simulink model "gm_UZ_D_GaN_Inverter_reduced"  (R2020b)
settings: Solver=FixedStepDiscrete  StartTime=0.0  StopTime=300e-6  RelTol=1e-3
libraries: simulink x24, hdlsllib x6
settings Model: Creator=Michael Hoerner  LastModifiedBy=micha
settings DataIOCC: LimitDataPoints=on  SaveOutput=off  SaveTime=off
settings OptimizationCC: BlockReduction=off  ConditionallyExecuteInputs=off  DefaultParameterBehavior=Inlined  LifeSpan=inf
settings DebuggingCC: AlgebraicLoopMsg=error  InheritedTsInSrcMsg=none  SingleTaskRateTransMsg=error  AllowSymbolicDim=off  StrictBusMsg=ErrorOnBusTreatedAsVector  SFUnexpectedBacktrackingDiag=warning  SFNoUnconditionalDefaultTransitionDiag=warning  SFExecutionAtInitializationDiag=none  ArithmeticOperatorsInVariantConditions=warning
settings HardwareCC: ProdBitPerPointer=32  ProdBitPerSizeT=32  ProdBitPerPtrDiffT=32  ProdLargestAtomicFloat=None  ProdIntDivRoundTo=Undefined  ProdEndianess=Unspecified  ProdWordSize=32  ProdHWDeviceType=ASIC/FPGA->ASIC/FPGA  ProdEqTarget=off
settings SFSimCC: SimUseLocalCustomCode=off  CustomCodeUndefinedFunction=UseInterfaceOnly
settings RTWCC: RTWUseLocalCustomCode=off
settings CodeAppCC: StateflowObjectComments=on
settings GRTTargetCC: TargetLangStandard=C89/C90 (ANSI)
settings ConfigComp: CovScope=ReferencedModels  CovMetricSettings=dw  CovSaveCumulativeToWorkspaceVar=on  CovSaveSingleToWorkspaceVar=on  CovExternalEMLEnable=off  CovSFcnEnable=off

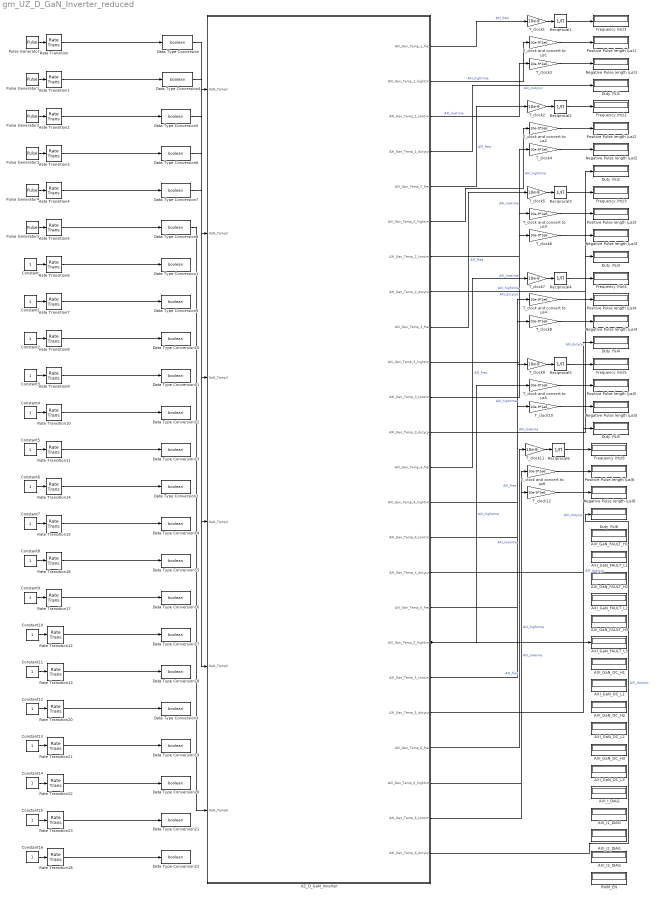
== system gm_UZ_D_GaN_Inverter_reduced ==
  AXI_GaN_FAULT_H1 : Display
  AXI_GaN_FAULT_H2 : Display
  AXI_GaN_FAULT_H3 : Display
  AXI_GaN_FAULT_L1 : Display
  AXI_GaN_FAULT_L2 : Display
  AXI_GaN_FAULT_L3 : Display
  AXI_GaN_OC_H1 : Display
  AXI_GaN_OC_H2 : Display
  AXI_GaN_OC_H3 : Display
  AXI_GaN_OC_L1 : Display
  AXI_GaN_OC_L2 : Display
  AXI_GaN_OC_L3 : Display
  AXI_I1_DIAG : Display
  AXI_I2_DIAG : Display
  AXI_I3_DIAG : Display
  AXI_I_DIAG : Display
  Constant{,1..16} (17 alike) : Constant
  Data Type Conversion{,1..22} (23 alike) : DataTypeConversion  OutDataTypeStr=boolean
  Duty (%){1..6} (6 alike) : Display
  Frequency (Hz){1..6} (6 alike) : Display
  Negative Pulse length (µs){1..6} (6 alike) : Display
  PWM_EN : Display
  Positive Pulse length (µs){1..6} (6 alike) : Display
  Pulse Generator : DiscretePulseGenerator  PulseType=Time based  Period=1/10000  PulseWidth=7
  Pulse Generator1 : DiscretePulseGenerator  PulseType=Time based  Period=1/10000  PulseWidth=8
  Pulse Generator2 : DiscretePulseGenerator  PulseType=Time based  Period=1/10000  PulseWidth=9
  Pulse Generator3 : DiscretePulseGenerator  PulseType=Time based  Period=1/10000  PulseWidth=10
  Pulse Generator4 : DiscretePulseGenerator  PulseType=Time based  Period=1/10000  PulseWidth=11
  Pulse Generator5 : DiscretePulseGenerator  PulseType=Time based  Period=1/10000  PulseWidth=12
  Rate Transition{,1..18,20..23} (23 alike) : RateTransition  OutPortSampleTime=10e-9
  Reciprocal{1..6} (6 alike) : Product  Inputs=/
  T_clock and convert to µs{1..6} (6 alike) : Gain  Gain=10e-9*1e6
  T_clock{1..2,5,7,9,11} (6 alike) : Gain  Gain=10e-9
  T_clock{3..4,6,8,10,12} (6 alike) : Gain  Gain=10e-9*1e6
  UZ_D_GaN_Inverter : Subsystem  TreatAsAtomicUnit=on
  wires:
  ? -> PWM_EN/1
  Rate Transition18/1 -> Data Type Conversion22/1
  Constant16/1 -> Rate Transition18/1
  Data Type Conversion8/1 -> UZ_D_GaN_Inverter/6(GaN_Temp6)
  Data Type Conversion7/1 -> UZ_D_GaN_Inverter/5(GaN_Temp5)
  Data Type Conversion6/1 -> UZ_D_GaN_Inverter/4(GaN_Temp4)
  Data Type Conversion5/1 -> UZ_D_GaN_Inverter/3(GaN_Temp3)
  Data Type Conversion4/1 -> UZ_D_GaN_Inverter/2(GaN_Temp2)
  ? -> AXI_I3_DIAG/1
  ? -> AXI_I2_DIAG/1
  ? -> AXI_I1_DIAG/1
  ? -> AXI_I_DIAG/1
  ? -> AXI_GaN_OC_L3/1
  ? -> AXI_GaN_OC_H3/1
  ? -> AXI_GaN_OC_L2/1
  ? -> AXI_GaN_OC_H2/1
  ? -> AXI_GaN_OC_L1/1
  ? -> AXI_GaN_OC_H1/1
  UZ_D_GaN_Inverter/18(AXI_Gan_Temp_5_hightime) -> AXI_GaN_FAULT_L3/1, T_clock and convert to µs5/1  "AXI_hightime"
  ? -> AXI_GaN_FAULT_H3/1
  ? -> AXI_GaN_FAULT_L2/1
  ? -> AXI_GaN_FAULT_H2/1
  ? -> AXI_GaN_FAULT_L1/1
  ? -> AXI_GaN_FAULT_H1/1
  UZ_D_GaN_Inverter/21(AXI_Gan_Temp_6_freq) -> T_clock11/1  "AXI_freq"
  T_clock and convert to µs6/1 -> Positive Pulse length (µs)6/1
  UZ_D_GaN_Inverter/22(AXI_Gan_Temp_6_hightime) -> T_clock and convert to µs6/1  "AXI_hightime"
  T_clock12/1 -> Negative Pulse length (µs)6/1
  Reciprocal6/1 -> Frequency (Hz)6/1
  UZ_D_GaN_Inverter/24(AXI_Gan_Temp_6_dutycyc) -> Duty (%)6/1  "AXI_dutycyc"
  T_clock11/1 -> Reciprocal6/1
  UZ_D_GaN_Inverter/23(AXI_Gan_Temp_6_lowtime) -> T_clock12/1  "AXI_lowtime"
  UZ_D_GaN_Inverter/17(AXI_Gan_Temp_5_freq) -> T_clock9/1  "AXI_freq"
  T_clock and convert to µs5/1 -> Positive Pulse length (µs)5/1
  T_clock10/1 -> Negative Pulse length (µs)5/1
  Reciprocal5/1 -> Frequency (Hz)5/1
  UZ_D_GaN_Inverter/20(AXI_Gan_Temp_5_dutycyc) -> Duty (%)5/1  "AXI_dutycyc"
  T_clock9/1 -> Reciprocal5/1
  UZ_D_GaN_Inverter/19(AXI_Gan_Temp_5_lowtime) -> T_clock10/1  "AXI_lowtime"
  UZ_D_GaN_Inverter/13(AXI_Gan_Temp_4_freq) -> T_clock7/1  "AXI_freq"
  T_clock and convert to µs4/1 -> Positive Pulse length (µs)4/1
  UZ_D_GaN_Inverter/14(AXI_Gan_Temp_4_hightime) -> T_clock and convert to µs4/1  "AXI_hightime"
  T_clock8/1 -> Negative Pulse length (µs)4/1
  Reciprocal4/1 -> Frequency (Hz)4/1
  UZ_D_GaN_Inverter/16(AXI_Gan_Temp_4_dutycyc) -> Duty (%)4/1  "AXI_dutycyc"
  T_clock7/1 -> Reciprocal4/1
  UZ_D_GaN_Inverter/15(AXI_Gan_Temp_4_lowtime) -> T_clock8/1  "AXI_lowtime"
  UZ_D_GaN_Inverter/9(AXI_Gan_Temp_3_freq) -> T_clock5/1  "AXI_freq"
  T_clock and convert to µs3/1 -> Positive Pulse length (µs)3/1
  UZ_D_GaN_Inverter/10(AXI_Gan_Temp_3_hightime) -> T_clock and convert to µs3/1  "AXI_hightime"
  T_clock6/1 -> Negative Pulse length (µs)3/1
  Reciprocal3/1 -> Frequency (Hz)3/1
  UZ_D_GaN_Inverter/12(AXI_Gan_Temp_3_dutycyc) -> Duty (%)3/1  "AXI_dutycyc"
  T_clock5/1 -> Reciprocal3/1
  UZ_D_GaN_Inverter/11(AXI_Gan_Temp_3_lowtime) -> T_clock6/1  "AXI_lowtime"
  UZ_D_GaN_Inverter/5(AXI_Gan_Temp_2_freq) -> T_clock2/1  "AXI_freq"
  T_clock and convert to µs2/1 -> Positive Pulse length (µs)2/1
  UZ_D_GaN_Inverter/6(AXI_Gan_Temp_2_hightime) -> T_clock and convert to µs2/1  "AXI_hightime"
  T_clock4/1 -> Negative Pulse length (µs)2/1
  Reciprocal2/1 -> Frequency (Hz)2/1
  UZ_D_GaN_Inverter/8(AXI_Gan_Temp_2_dutycyc) -> Duty (%)2/1  "AXI_dutycyc"
  T_clock2/1 -> Reciprocal2/1
  UZ_D_GaN_Inverter/7(AXI_Gan_Temp_2_lowtime) -> T_clock4/1  "AXI_lowtime"
  UZ_D_GaN_Inverter/4(AXI_Gan_Temp_1_dutycyc) -> Duty (%)1/1  "AXI_dutycyc"
  UZ_D_GaN_Inverter/1(AXI_Gan_Temp_1_freq) -> T_clock1/1  "AXI_freq"
  T_clock1/1 -> Reciprocal1/1
  UZ_D_GaN_Inverter/2(AXI_Gan_Temp_1_hightime) -> T_clock and convert to µs1/1  "AXI_hightime"
  UZ_D_GaN_Inverter/3(AXI_Gan_Temp_1_lowtime) -> T_clock3/1  "AXI_lowtime"
  Reciprocal1/1 -> Frequency (Hz)1/1
  T_clock3/1 -> Negative Pulse length (µs)1/1
  T_clock and convert to µs1/1 -> Positive Pulse length (µs)1/1
  Constant12/1 -> Rate Transition20/1
  Constant14/1 -> Rate Transition22/1
  Constant13/1 -> Rate Transition21/1
  Constant15/1 -> Rate Transition23/1
  Constant6/1 -> Rate Transition14/1
  Constant11/1 -> Rate Transition13/1
  Constant8/1 -> Rate Transition16/1
  Constant10/1 -> Rate Transition12/1
  Constant7/1 -> Rate Transition15/1
  Constant9/1 -> Rate Transition17/1
  Constant5/1 -> Rate Transition11/1
  Constant4/1 -> Rate Transition10/1
  Constant3/1 -> Rate Transition9/1
  Constant2/1 -> Rate Transition8/1
  Constant1/1 -> Rate Transition7/1
  Constant/1 -> Rate Transition6/1
  Rate Transition22/1 -> Data Type Conversion20/1
  Rate Transition23/1 -> Data Type Conversion21/1
  Rate Transition21/1 -> Data Type Conversion19/1
  Rate Transition20/1 -> Data Type Conversion3/1
  Rate Transition16/1 -> Data Type Conversion15/1
  Rate Transition13/1 -> Data Type Conversion18/1
  Rate Transition17/1 -> Data Type Conversion16/1
  Rate Transition15/1 -> Data Type Conversion14/1
  Rate Transition14/1 -> Data Type Conversion2/1
  Rate Transition12/1 -> Data Type Conversion17/1
  Rate Transition7/1 -> Data Type Conversion9/1
  Rate Transition8/1 -> Data Type Conversion10/1
  Rate Transition10/1 -> Data Type Conversion12/1
  Rate Transition6/1 -> Data Type Conversion1/1
  Rate Transition11/1 -> Data Type Conversion13/1
  Rate Transition9/1 -> Data Type Conversion11/1
  Rate Transition5/1 -> Data Type Conversion8/1
  Rate Transition4/1 -> Data Type Conversion7/1
  Rate Transition3/1 -> Data Type Conversion6/1
  Rate Transition2/1 -> Data Type Conversion5/1
  Rate Transition1/1 -> Data Type Conversion4/1
  Rate Transition/1 -> Data Type Conversion/1
  Pulse Generator5/1 -> Rate Transition5/1
  Pulse Generator4/1 -> Rate Transition4/1
  Pulse Generator3/1 -> Rate Transition3/1
  Pulse Generator2/1 -> Rate Transition2/1
  Pulse Generator1/1 -> Rate Transition1/1
  Pulse Generator/1 -> Rate Transition/1
  Data Type Conversion/1 -> UZ_D_GaN_Inverter/1(GaN_Temp1)

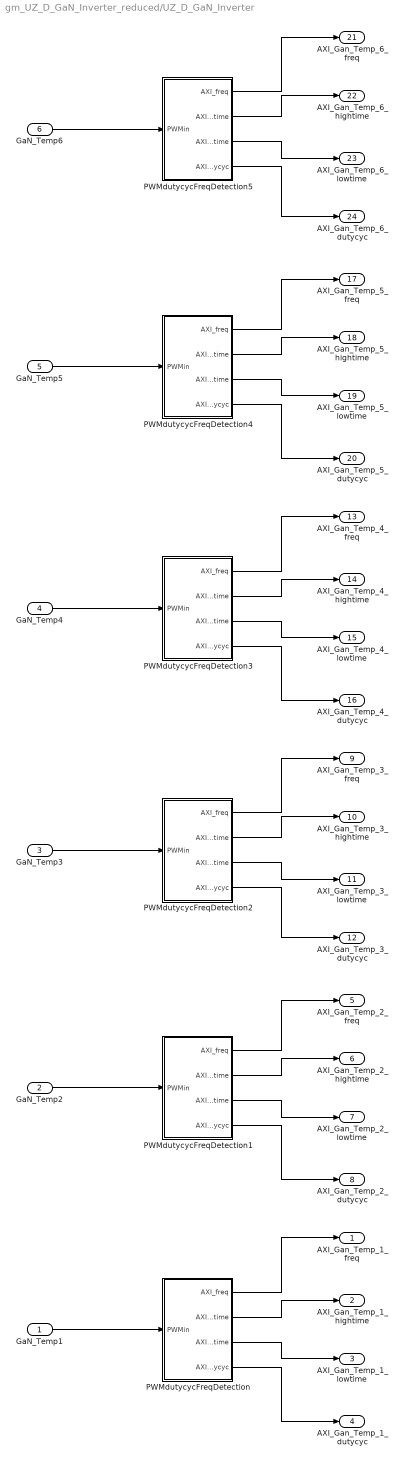
== system gm_UZ_D_GaN_Inverter_reduced/UZ_D_GaN_Inverter ==
  GaN_Temp1 : Inport  OutDataTypeStr=boolean  PortDimensions=1  SampleTime=1e-08
  GaN_Temp2 : Inport  Port=2  OutDataTypeStr=boolean  PortDimensions=1  SampleTime=1e-08
  GaN_Temp3 : Inport  Port=3  OutDataTypeStr=boolean  PortDimensions=1  SampleTime=1e-08
  GaN_Temp4 : Inport  Port=4  OutDataTypeStr=boolean  PortDimensions=1  SampleTime=1e-08
  GaN_Temp5 : Inport  Port=5  OutDataTypeStr=boolean  PortDimensions=1  SampleTime=1e-08
  GaN_Temp6 : Inport  Port=6  OutDataTypeStr=boolean  PortDimensions=1  SampleTime=1e-08
  PWMdutycycFreqDetection : Subsystem
  PWMdutycycFreqDetection1 : Subsystem
  PWMdutycycFreqDetection2 : Subsystem
  PWMdutycycFreqDetection3 : Subsystem
  PWMdutycycFreqDetection4 : Subsystem
  PWMdutycycFreqDetection5 : Subsystem
  AXI_Gan_Temp_1_freq : Outport  PortDimensions=1  VectorParamsAs1DForOutWhenUnconnected=off
  AXI_Gan_Temp_1_hightime : Outport  Port=2  PortDimensions=1  VectorParamsAs1DForOutWhenUnconnected=off
  AXI_Gan_Temp_1_lowtime : Outport  Port=3  PortDimensions=1  VectorParamsAs1DForOutWhenUnconnected=off
  AXI_Gan_Temp_1_dutycyc : Outport  Port=4  PortDimensions=1  VectorParamsAs1DForOutWhenUnconnected=off
  AXI_Gan_Temp_2_freq : Outport  Port=5  PortDimensions=1  VectorParamsAs1DForOutWhenUnconnected=off
  AXI_Gan_Temp_2_hightime : Outport  Port=6  PortDimensions=1  VectorParamsAs1DForOutWhenUnconnected=off
  AXI_Gan_Temp_2_lowtime : Outport  Port=7  PortDimensions=1  VectorParamsAs1DForOutWhenUnconnected=off
  AXI_Gan_Temp_2_dutycyc : Outport  Port=8  PortDimensions=1  VectorParamsAs1DForOutWhenUnconnected=off
  AXI_Gan_Temp_3_freq : Outport  Port=9  PortDimensions=1  VectorParamsAs1DForOutWhenUnconnected=off
  AXI_Gan_Temp_3_hightime : Outport  Port=10  PortDimensions=1  VectorParamsAs1DForOutWhenUnconnected=off
  AXI_Gan_Temp_3_lowtime : Outport  Port=11  PortDimensions=1  VectorParamsAs1DForOutWhenUnconnected=off
  AXI_Gan_Temp_3_dutycyc : Outport  Port=12  PortDimensions=1  VectorParamsAs1DForOutWhenUnconnected=off
  AXI_Gan_Temp_4_freq : Outport  Port=13  PortDimensions=1  VectorParamsAs1DForOutWhenUnconnected=off
  AXI_Gan_Temp_4_hightime : Outport  Port=14  PortDimensions=1  VectorParamsAs1DForOutWhenUnconnected=off
  AXI_Gan_Temp_4_lowtime : Outport  Port=15  PortDimensions=1  VectorParamsAs1DForOutWhenUnconnected=off
  AXI_Gan_Temp_4_dutycyc : Outport  Port=16  PortDimensions=1  VectorParamsAs1DForOutWhenUnconnected=off
  AXI_Gan_Temp_5_freq : Outport  Port=17  PortDimensions=1  VectorParamsAs1DForOutWhenUnconnected=off
  AXI_Gan_Temp_5_hightime : Outport  Port=18  PortDimensions=1  VectorParamsAs1DForOutWhenUnconnected=off
  AXI_Gan_Temp_5_lowtime : Outport  Port=19  PortDimensions=1  VectorParamsAs1DForOutWhenUnconnected=off
  AXI_Gan_Temp_5_dutycyc : Outport  Port=20  PortDimensions=1  VectorParamsAs1DForOutWhenUnconnected=off
  AXI_Gan_Temp_6_freq : Outport  Port=21  PortDimensions=1  VectorParamsAs1DForOutWhenUnconnected=off
  AXI_Gan_Temp_6_hightime : Outport  Port=22  PortDimensions=1  VectorParamsAs1DForOutWhenUnconnected=off
  AXI_Gan_Temp_6_lowtime : Outport  Port=23  PortDimensions=1  VectorParamsAs1DForOutWhenUnconnected=off
  AXI_Gan_Temp_6_dutycyc : Outport  Port=24  PortDimensions=1  VectorParamsAs1DForOutWhenUnconnected=off
  wires:
  GaN_Temp1/1 -> PWMdutycycFreqDetection/1(PWMin)
  GaN_Temp2/1 -> PWMdutycycFreqDetection1/1(PWMin)
  GaN_Temp3/1 -> PWMdutycycFreqDetection2/1(PWMin)
  GaN_Temp4/1 -> PWMdutycycFreqDetection3/1(PWMin)
  GaN_Temp5/1 -> PWMdutycycFreqDetection4/1(PWMin)
  GaN_Temp6/1 -> PWMdutycycFreqDetection5/1(PWMin)
  PWMdutycycFreqDetection/1(AXI_freq) -> AXI_Gan_Temp_1_freq/1
  PWMdutycycFreqDetection/2(AXI_hightime) -> AXI_Gan_Temp_1_hightime/1
  PWMdutycycFreqDetection/3(AXI_lowtime) -> AXI_Gan_Temp_1_lowtime/1
  PWMdutycycFreqDetection/4(AXI_dutycyc) -> AXI_Gan_Temp_1_dutycyc/1
  PWMdutycycFreqDetection1/1(AXI_freq) -> AXI_Gan_Temp_2_freq/1
  PWMdutycycFreqDetection1/2(AXI_hightime) -> AXI_Gan_Temp_2_hightime/1
  PWMdutycycFreqDetection1/3(AXI_lowtime) -> AXI_Gan_Temp_2_lowtime/1
  PWMdutycycFreqDetection1/4(AXI_dutycyc) -> AXI_Gan_Temp_2_dutycyc/1
  PWMdutycycFreqDetection2/1(AXI_freq) -> AXI_Gan_Temp_3_freq/1
  PWMdutycycFreqDetection2/2(AXI_hightime) -> AXI_Gan_Temp_3_hightime/1
  PWMdutycycFreqDetection2/3(AXI_lowtime) -> AXI_Gan_Temp_3_lowtime/1
  PWMdutycycFreqDetection2/4(AXI_dutycyc) -> AXI_Gan_Temp_3_dutycyc/1
  PWMdutycycFreqDetection3/1(AXI_freq) -> AXI_Gan_Temp_4_freq/1
  PWMdutycycFreqDetection3/2(AXI_hightime) -> AXI_Gan_Temp_4_hightime/1
  PWMdutycycFreqDetection3/3(AXI_lowtime) -> AXI_Gan_Temp_4_lowtime/1
  PWMdutycycFreqDetection3/4(AXI_dutycyc) -> AXI_Gan_Temp_4_dutycyc/1
  PWMdutycycFreqDetection4/1(AXI_freq) -> AXI_Gan_Temp_5_freq/1
  PWMdutycycFreqDetection4/2(AXI_hightime) -> AXI_Gan_Temp_5_hightime/1
  PWMdutycycFreqDetection4/3(AXI_lowtime) -> AXI_Gan_Temp_5_lowtime/1
  PWMdutycycFreqDetection4/4(AXI_dutycyc) -> AXI_Gan_Temp_5_dutycyc/1
  PWMdutycycFreqDetection5/1(AXI_freq) -> AXI_Gan_Temp_6_freq/1
  PWMdutycycFreqDetection5/2(AXI_hightime) -> AXI_Gan_Temp_6_hightime/1
  PWMdutycycFreqDetection5/3(AXI_lowtime) -> AXI_Gan_Temp_6_lowtime/1
  PWMdutycycFreqDetection5/4(AXI_dutycyc) -> AXI_Gan_Temp_6_dutycyc/1

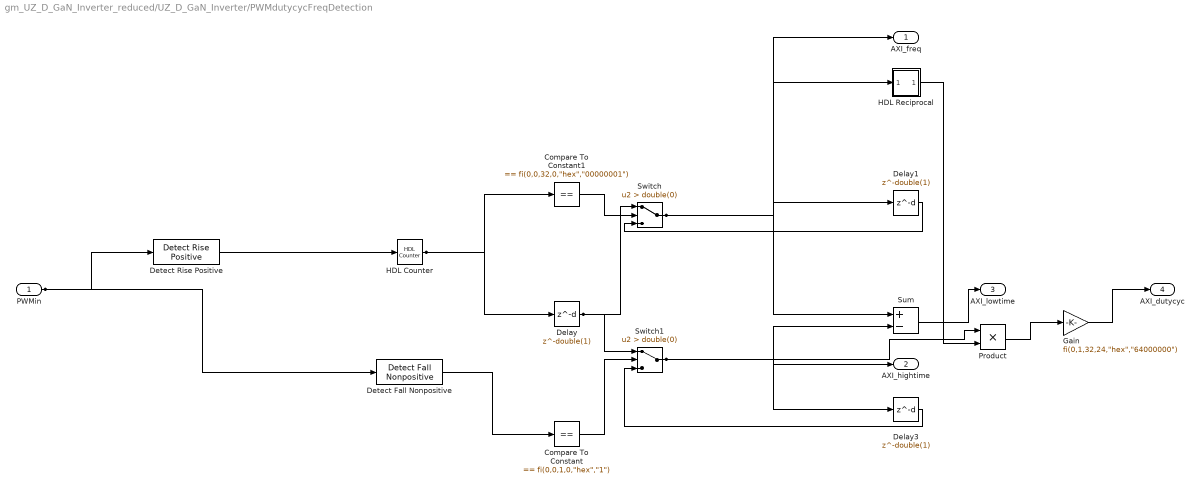
== system gm_UZ_D_GaN_Inverter_reduced/UZ_D_GaN_Inverter/PWMdutycycFreqDetection ==
  PWMin : Inport  OutDataTypeStr=boolean  PortDimensions=1  SampleTime=1e-08
  Compare To Constant : simulink/Logic and Bit Operations/Compare To Constant  relop===  const="fi(0,0,1,0,\"hex\",\"1\")"  OutDataTypeStr=boolean
  Compare To Constant1 : simulink/Logic and Bit Operations/Compare To Constant  relop===  const="fi(0,0,32,0,\"hex\",\"00000001\")"  OutDataTypeStr=boolean
  Delay : Delay  DelayLength=double(1)  InitialCondition=0  SampleTime=1e-08
  Delay1 : Delay  DelayLength=double(1)  InitialCondition=0  SampleTime=1e-08
  Delay3 : Delay  DelayLength=double(1)  InitialCondition=0  SampleTime=1e-08
  Detect Fall Nonpositive : simulink/Logic and Bit Operations/Detect Fall Nonpositive  vinit=0  OutDataTypeStr=boolean
      settings: SourceProductBaseCode=SL
  Detect Rise Positive : simulink/Logic and Bit Operations/Detect Rise Positive  vinit=0  OutDataTypeStr=boolean
  Gain : Gain  Gain="fi(0,1,32,24,\"hex\",\"64000000\")"  ParamDataTypeStr=fixdt(1, 32, 24)  OutDataTypeStr=fixdt(1, 32, 24)  SampleTime=1e-08
  HDL Counter : hdlsllib/Sources/HDL Counter  CountType=Count limited  CountInit=double(1)  CountStep=double(1)  CountMax=double(2500000)  CountFromType=Initial value  CountFrom=double(1)  CountResetPort=on  CountLoadPort=off  CountEnbPort=off  CountDirPort=off  CountDataType=Unsigned  CountWordLen=32  CountFracLen=0  CountSampTime=1e-08
  HDL Reciprocal : Subsystem
  Product : Product  Inputs=**  OutDataTypeStr=fixdt(1, 32, 30)  SampleTime=1e-08
  Sum : Sum  Inputs=+-  AccumDataTypeStr=uint32  OutDataTypeStr=uint32  SampleTime=1e-08
  Switch : Switch  Criteria=u2 > Threshold  Threshold=double(0)  OutDataTypeStr=uint32  SampleTime=1e-08
  Switch1 : Switch  Criteria=u2 > Threshold  Threshold=double(0)  OutDataTypeStr=uint32  SampleTime=1e-08
  AXI_freq : Outport  VectorParamsAs1DForOutWhenUnconnected=off
  AXI_hightime : Outport  Port=2  VectorParamsAs1DForOutWhenUnconnected=off
  AXI_lowtime : Outport  Port=3  VectorParamsAs1DForOutWhenUnconnected=off
  AXI_dutycyc : Outport  Port=4  VectorParamsAs1DForOutWhenUnconnected=off
  wires:
  PWMin/1 -> Detect Fall Nonpositive/1, Detect Rise Positive/1
  Compare To Constant/1 -> Switch1/2
  Compare To Constant1/1 -> Switch/2
  Delay/1 -> Switch/1, Switch1/1
  Detect Fall Nonpositive/1 -> Compare To Constant/1
  Detect Rise Positive/1 -> HDL Counter/1
  Gain/1 -> AXI_dutycyc/1
  HDL Counter/1 -> Compare To Constant1/1, Delay/1
  HDL Reciprocal/1(Out1) -> Product/2
  Product/1 -> Gain/1
  Sum/1 -> AXI_lowtime/1
  Switch/1 -> Sum/1, HDL Reciprocal/1(In1), AXI_freq/1, Delay1/1
  Switch1/1 -> Sum/2, Product/1, AXI_hightime/1, Delay3/1
  Delay1/1 -> Switch/3
  Delay3/1 -> Switch1/3

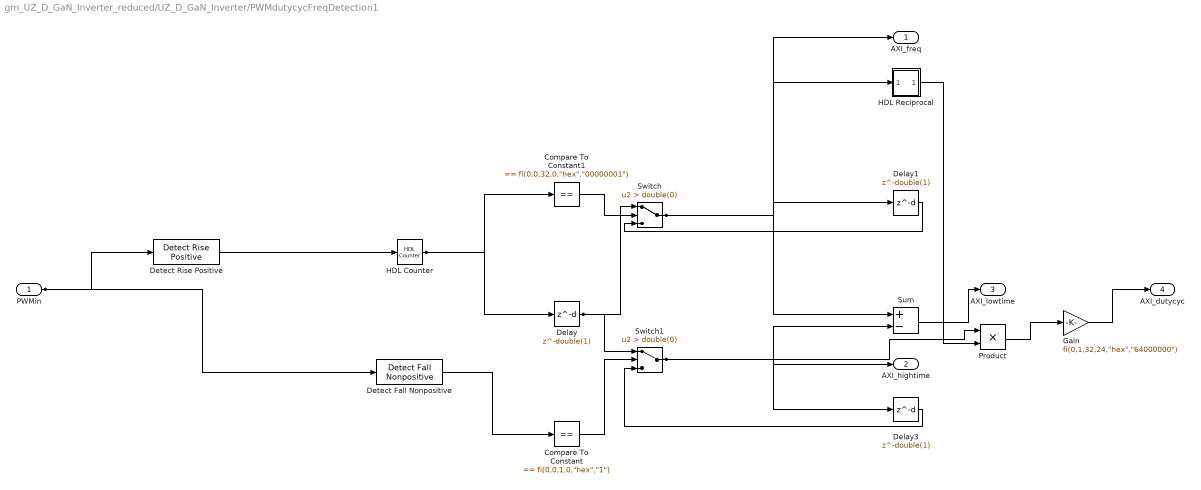
== system gm_UZ_D_GaN_Inverter_reduced/UZ_D_GaN_Inverter/PWMdutycycFreqDetection1 ==
  PWMin : Inport  OutDataTypeStr=boolean  PortDimensions=1  SampleTime=1e-08
  Compare To Constant : simulink/Logic and Bit Operations/Compare To Constant  relop===  const="fi(0,0,1,0,\"hex\",\"1\")"  OutDataTypeStr=boolean
  Compare To Constant1 : simulink/Logic and Bit Operations/Compare To Constant  relop===  const="fi(0,0,32,0,\"hex\",\"00000001\")"  OutDataTypeStr=boolean
  Delay : Delay  DelayLength=double(1)  InitialCondition=0  SampleTime=1e-08
  Delay1 : Delay  DelayLength=double(1)  InitialCondition=0  SampleTime=1e-08
  Delay3 : Delay  DelayLength=double(1)  InitialCondition=0  SampleTime=1e-08
  Detect Fall Nonpositive : simulink/Logic and Bit Operations/Detect Fall Nonpositive  vinit=0  OutDataTypeStr=boolean
      settings: SourceProductBaseCode=SL
  Detect Rise Positive : simulink/Logic and Bit Operations/Detect Rise Positive  vinit=0  OutDataTypeStr=boolean
  Gain : Gain  Gain="fi(0,1,32,24,\"hex\",\"64000000\")"  ParamDataTypeStr=fixdt(1, 32, 24)  OutDataTypeStr=fixdt(1, 32, 24)  SampleTime=1e-08
  HDL Counter : hdlsllib/Sources/HDL Counter  CountType=Count limited  CountInit=double(1)  CountStep=double(1)  CountMax=double(2500000)  CountFromType=Initial value  CountFrom=double(1)  CountResetPort=on  CountLoadPort=off  CountEnbPort=off  CountDirPort=off  CountDataType=Unsigned  CountWordLen=32  CountFracLen=0  CountSampTime=1e-08
  HDL Reciprocal : Subsystem
  Product : Product  Inputs=**  OutDataTypeStr=fixdt(1, 32, 30)  SampleTime=1e-08
  Sum : Sum  Inputs=+-  AccumDataTypeStr=uint32  OutDataTypeStr=uint32  SampleTime=1e-08
  Switch : Switch  Criteria=u2 > Threshold  Threshold=double(0)  OutDataTypeStr=uint32  SampleTime=1e-08
  Switch1 : Switch  Criteria=u2 > Threshold  Threshold=double(0)  OutDataTypeStr=uint32  SampleTime=1e-08
  AXI_freq : Outport  VectorParamsAs1DForOutWhenUnconnected=off
  AXI_hightime : Outport  Port=2  VectorParamsAs1DForOutWhenUnconnected=off
  AXI_lowtime : Outport  Port=3  VectorParamsAs1DForOutWhenUnconnected=off
  AXI_dutycyc : Outport  Port=4  VectorParamsAs1DForOutWhenUnconnected=off
  wires:
  Delay3/1 -> Switch1/3
  Delay1/1 -> Switch/3
  Switch1/1 -> Delay3/1, AXI_hightime/1, Product/1, Sum/2
  Switch/1 -> Delay1/1, AXI_freq/1, HDL Reciprocal/1(In1), Sum/1
  Sum/1 -> AXI_lowtime/1
  Product/1 -> Gain/1
  HDL Reciprocal/1(Out1) -> Product/2
  HDL Counter/1 -> Delay/1, Compare To Constant1/1
  Gain/1 -> AXI_dutycyc/1
  Detect Rise Positive/1 -> HDL Counter/1
  Detect Fall Nonpositive/1 -> Compare To Constant/1
  Delay/1 -> Switch1/1, Switch/1
  Compare To Constant1/1 -> Switch/2
  Compare To Constant/1 -> Switch1/2
  PWMin/1 -> Detect Rise Positive/1, Detect Fall Nonpositive/1

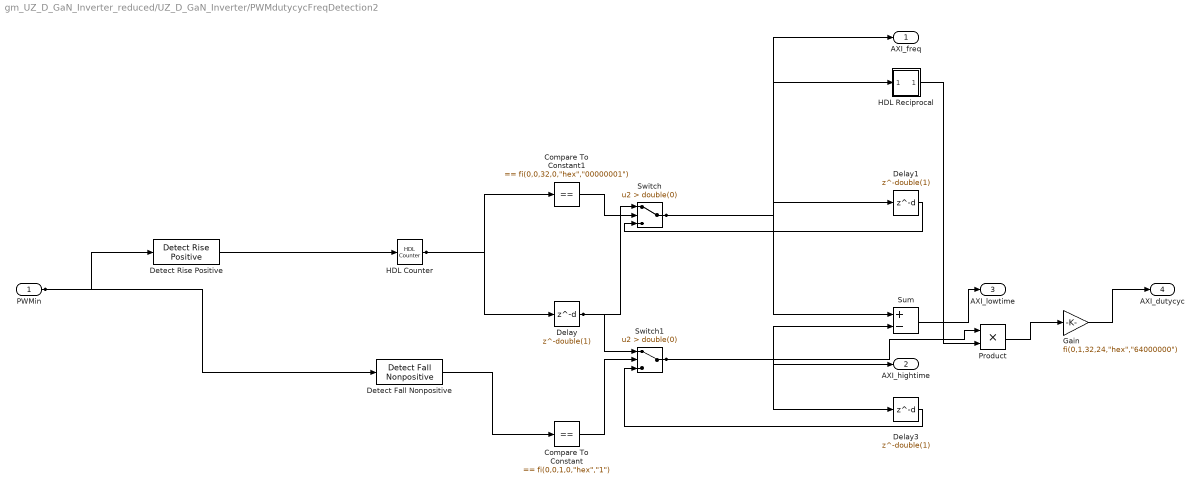
== system gm_UZ_D_GaN_Inverter_reduced/UZ_D_GaN_Inverter/PWMdutycycFreqDetection2 ==
  PWMin : Inport  OutDataTypeStr=boolean  PortDimensions=1  SampleTime=1e-08
  Compare To Constant : simulink/Logic and Bit Operations/Compare To Constant  relop===  const="fi(0,0,1,0,\"hex\",\"1\")"  OutDataTypeStr=boolean
  Compare To Constant1 : simulink/Logic and Bit Operations/Compare To Constant  relop===  const="fi(0,0,32,0,\"hex\",\"00000001\")"  OutDataTypeStr=boolean
  Delay : Delay  DelayLength=double(1)  InitialCondition=0  SampleTime=1e-08
  Delay1 : Delay  DelayLength=double(1)  InitialCondition=0  SampleTime=1e-08
  Delay3 : Delay  DelayLength=double(1)  InitialCondition=0  SampleTime=1e-08
  Detect Fall Nonpositive : simulink/Logic and Bit Operations/Detect Fall Nonpositive  vinit=0  OutDataTypeStr=boolean
      settings: SourceProductBaseCode=SL
  Detect Rise Positive : simulink/Logic and Bit Operations/Detect Rise Positive  vinit=0  OutDataTypeStr=boolean
  Gain : Gain  Gain="fi(0,1,32,24,\"hex\",\"64000000\")"  ParamDataTypeStr=fixdt(1, 32, 24)  OutDataTypeStr=fixdt(1, 32, 24)  SampleTime=1e-08
  HDL Counter : hdlsllib/Sources/HDL Counter  CountType=Count limited  CountInit=double(1)  CountStep=double(1)  CountMax=double(2500000)  CountFromType=Initial value  CountFrom=double(1)  CountResetPort=on  CountLoadPort=off  CountEnbPort=off  CountDirPort=off  CountDataType=Unsigned  CountWordLen=32  CountFracLen=0  CountSampTime=1e-08
  HDL Reciprocal : Subsystem
  Product : Product  Inputs=**  OutDataTypeStr=fixdt(1, 32, 30)  SampleTime=1e-08
  Sum : Sum  Inputs=+-  AccumDataTypeStr=uint32  OutDataTypeStr=uint32  SampleTime=1e-08
  Switch : Switch  Criteria=u2 > Threshold  Threshold=double(0)  OutDataTypeStr=uint32  SampleTime=1e-08
  Switch1 : Switch  Criteria=u2 > Threshold  Threshold=double(0)  OutDataTypeStr=uint32  SampleTime=1e-08
  AXI_freq : Outport  VectorParamsAs1DForOutWhenUnconnected=off
  AXI_hightime : Outport  Port=2  VectorParamsAs1DForOutWhenUnconnected=off
  AXI_lowtime : Outport  Port=3  VectorParamsAs1DForOutWhenUnconnected=off
  AXI_dutycyc : Outport  Port=4  VectorParamsAs1DForOutWhenUnconnected=off
  wires:
  Delay3/1 -> Switch1/3
  Delay1/1 -> Switch/3
  Switch1/1 -> Delay3/1, AXI_hightime/1, Product/1, Sum/2
  Switch/1 -> Delay1/1, AXI_freq/1, HDL Reciprocal/1(In1), Sum/1
  Sum/1 -> AXI_lowtime/1
  Product/1 -> Gain/1
  HDL Reciprocal/1(Out1) -> Product/2
  HDL Counter/1 -> Delay/1, Compare To Constant1/1
  Gain/1 -> AXI_dutycyc/1
  Detect Rise Positive/1 -> HDL Counter/1
  Detect Fall Nonpositive/1 -> Compare To Constant/1
  Delay/1 -> Switch1/1, Switch/1
  Compare To Constant1/1 -> Switch/2
  Compare To Constant/1 -> Switch1/2
  PWMin/1 -> Detect Rise Positive/1, Detect Fall Nonpositive/1

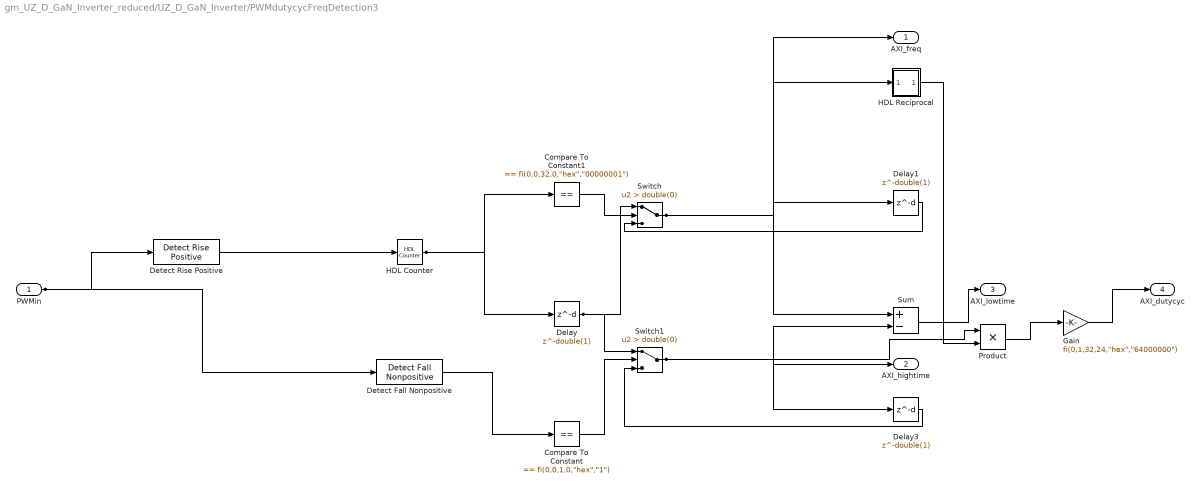
== system gm_UZ_D_GaN_Inverter_reduced/UZ_D_GaN_Inverter/PWMdutycycFreqDetection3 ==
  PWMin : Inport  OutDataTypeStr=boolean  PortDimensions=1  SampleTime=1e-08
  Compare To Constant : simulink/Logic and Bit Operations/Compare To Constant  relop===  const="fi(0,0,1,0,\"hex\",\"1\")"  OutDataTypeStr=boolean
  Compare To Constant1 : simulink/Logic and Bit Operations/Compare To Constant  relop===  const="fi(0,0,32,0,\"hex\",\"00000001\")"  OutDataTypeStr=boolean
  Delay : Delay  DelayLength=double(1)  InitialCondition=0  SampleTime=1e-08
  Delay1 : Delay  DelayLength=double(1)  InitialCondition=0  SampleTime=1e-08
  Delay3 : Delay  DelayLength=double(1)  InitialCondition=0  SampleTime=1e-08
  Detect Fall Nonpositive : simulink/Logic and Bit Operations/Detect Fall Nonpositive  vinit=0  OutDataTypeStr=boolean
      settings: SourceProductBaseCode=SL
  Detect Rise Positive : simulink/Logic and Bit Operations/Detect Rise Positive  vinit=0  OutDataTypeStr=boolean
  Gain : Gain  Gain="fi(0,1,32,24,\"hex\",\"64000000\")"  ParamDataTypeStr=fixdt(1, 32, 24)  OutDataTypeStr=fixdt(1, 32, 24)  SampleTime=1e-08
  HDL Counter : hdlsllib/Sources/HDL Counter  CountType=Count limited  CountInit=double(1)  CountStep=double(1)  CountMax=double(2500000)  CountFromType=Initial value  CountFrom=double(1)  CountResetPort=on  CountLoadPort=off  CountEnbPort=off  CountDirPort=off  CountDataType=Unsigned  CountWordLen=32  CountFracLen=0  CountSampTime=1e-08
  HDL Reciprocal : Subsystem
  Product : Product  Inputs=**  OutDataTypeStr=fixdt(1, 32, 30)  SampleTime=1e-08
  Sum : Sum  Inputs=+-  AccumDataTypeStr=uint32  OutDataTypeStr=uint32  SampleTime=1e-08
  Switch : Switch  Criteria=u2 > Threshold  Threshold=double(0)  OutDataTypeStr=uint32  SampleTime=1e-08
  Switch1 : Switch  Criteria=u2 > Threshold  Threshold=double(0)  OutDataTypeStr=uint32  SampleTime=1e-08
  AXI_freq : Outport  VectorParamsAs1DForOutWhenUnconnected=off
  AXI_hightime : Outport  Port=2  VectorParamsAs1DForOutWhenUnconnected=off
  AXI_lowtime : Outport  Port=3  VectorParamsAs1DForOutWhenUnconnected=off
  AXI_dutycyc : Outport  Port=4  VectorParamsAs1DForOutWhenUnconnected=off
  wires:
  Delay3/1 -> Switch1/3
  Delay1/1 -> Switch/3
  Switch1/1 -> Delay3/1, AXI_hightime/1, Product/1, Sum/2
  Switch/1 -> Delay1/1, AXI_freq/1, HDL Reciprocal/1(In1), Sum/1
  Sum/1 -> AXI_lowtime/1
  Product/1 -> Gain/1
  HDL Reciprocal/1(Out1) -> Product/2
  HDL Counter/1 -> Delay/1, Compare To Constant1/1
  Gain/1 -> AXI_dutycyc/1
  Detect Rise Positive/1 -> HDL Counter/1
  Detect Fall Nonpositive/1 -> Compare To Constant/1
  Delay/1 -> Switch1/1, Switch/1
  Compare To Constant1/1 -> Switch/2
  Compare To Constant/1 -> Switch1/2
  PWMin/1 -> Detect Rise Positive/1, Detect Fall Nonpositive/1

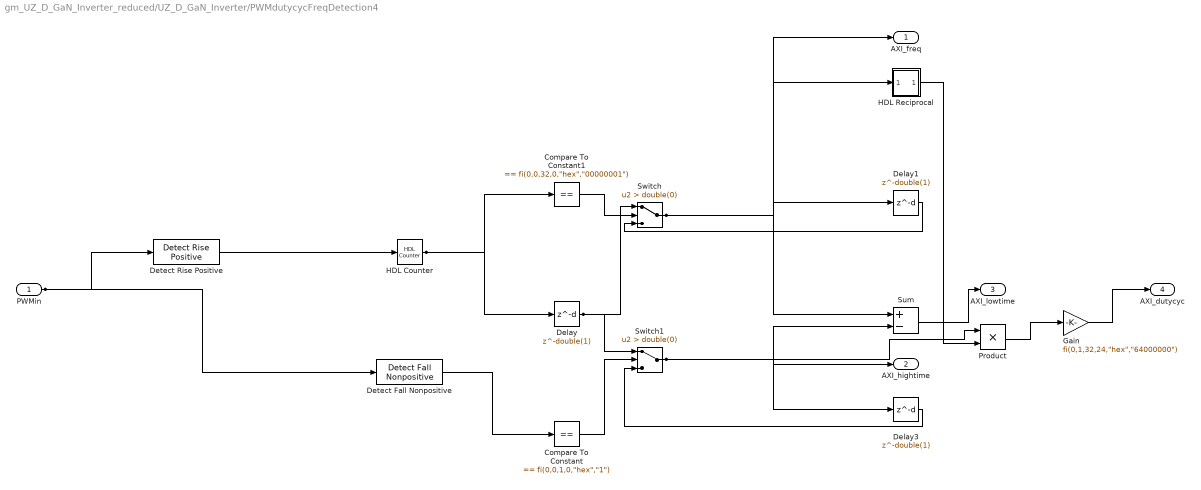
== system gm_UZ_D_GaN_Inverter_reduced/UZ_D_GaN_Inverter/PWMdutycycFreqDetection4 ==
  PWMin : Inport  OutDataTypeStr=boolean  PortDimensions=1  SampleTime=1e-08
  Compare To Constant : simulink/Logic and Bit Operations/Compare To Constant  relop===  const="fi(0,0,1,0,\"hex\",\"1\")"  OutDataTypeStr=boolean
  Compare To Constant1 : simulink/Logic and Bit Operations/Compare To Constant  relop===  const="fi(0,0,32,0,\"hex\",\"00000001\")"  OutDataTypeStr=boolean
  Delay : Delay  DelayLength=double(1)  InitialCondition=0  SampleTime=1e-08
  Delay1 : Delay  DelayLength=double(1)  InitialCondition=0  SampleTime=1e-08
  Delay3 : Delay  DelayLength=double(1)  InitialCondition=0  SampleTime=1e-08
  Detect Fall Nonpositive : simulink/Logic and Bit Operations/Detect Fall Nonpositive  vinit=0  OutDataTypeStr=boolean
      settings: SourceProductBaseCode=SL
  Detect Rise Positive : simulink/Logic and Bit Operations/Detect Rise Positive  vinit=0  OutDataTypeStr=boolean
  Gain : Gain  Gain="fi(0,1,32,24,\"hex\",\"64000000\")"  ParamDataTypeStr=fixdt(1, 32, 24)  OutDataTypeStr=fixdt(1, 32, 24)  SampleTime=1e-08
  HDL Counter : hdlsllib/Sources/HDL Counter  CountType=Count limited  CountInit=double(1)  CountStep=double(1)  CountMax=double(2500000)  CountFromType=Initial value  CountFrom=double(1)  CountResetPort=on  CountLoadPort=off  CountEnbPort=off  CountDirPort=off  CountDataType=Unsigned  CountWordLen=32  CountFracLen=0  CountSampTime=1e-08
  HDL Reciprocal : Subsystem
  Product : Product  Inputs=**  OutDataTypeStr=fixdt(1, 32, 30)  SampleTime=1e-08
  Sum : Sum  Inputs=+-  AccumDataTypeStr=uint32  OutDataTypeStr=uint32  SampleTime=1e-08
  Switch : Switch  Criteria=u2 > Threshold  Threshold=double(0)  OutDataTypeStr=uint32  SampleTime=1e-08
  Switch1 : Switch  Criteria=u2 > Threshold  Threshold=double(0)  OutDataTypeStr=uint32  SampleTime=1e-08
  AXI_freq : Outport  VectorParamsAs1DForOutWhenUnconnected=off
  AXI_hightime : Outport  Port=2  VectorParamsAs1DForOutWhenUnconnected=off
  AXI_lowtime : Outport  Port=3  VectorParamsAs1DForOutWhenUnconnected=off
  AXI_dutycyc : Outport  Port=4  VectorParamsAs1DForOutWhenUnconnected=off
  wires:
  Delay3/1 -> Switch1/3
  Delay1/1 -> Switch/3
  Switch1/1 -> Delay3/1, AXI_hightime/1, Product/1, Sum/2
  Switch/1 -> Delay1/1, AXI_freq/1, HDL Reciprocal/1(In1), Sum/1
  Sum/1 -> AXI_lowtime/1
  Product/1 -> Gain/1
  HDL Reciprocal/1(Out1) -> Product/2
  HDL Counter/1 -> Delay/1, Compare To Constant1/1
  Gain/1 -> AXI_dutycyc/1
  Detect Rise Positive/1 -> HDL Counter/1
  Detect Fall Nonpositive/1 -> Compare To Constant/1
  Delay/1 -> Switch1/1, Switch/1
  Compare To Constant1/1 -> Switch/2
  Compare To Constant/1 -> Switch1/2
  PWMin/1 -> Detect Rise Positive/1, Detect Fall Nonpositive/1

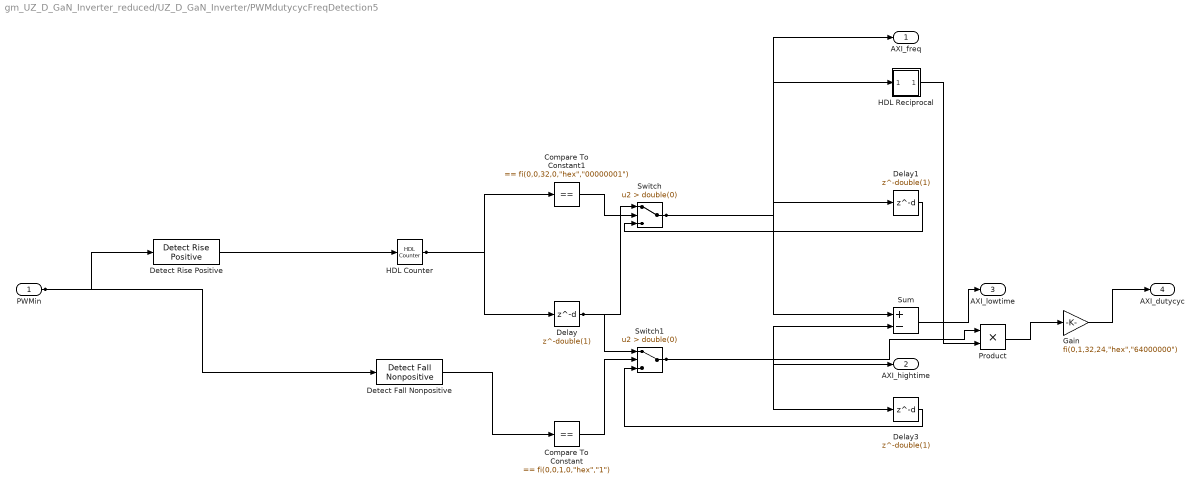
== system gm_UZ_D_GaN_Inverter_reduced/UZ_D_GaN_Inverter/PWMdutycycFreqDetection5 ==
  PWMin : Inport  OutDataTypeStr=boolean  PortDimensions=1  SampleTime=1e-08
  Compare To Constant : simulink/Logic and Bit Operations/Compare To Constant  relop===  const="fi(0,0,1,0,\"hex\",\"1\")"  OutDataTypeStr=boolean
  Compare To Constant1 : simulink/Logic and Bit Operations/Compare To Constant  relop===  const="fi(0,0,32,0,\"hex\",\"00000001\")"  OutDataTypeStr=boolean
  Delay : Delay  DelayLength=double(1)  InitialCondition=0  SampleTime=1e-08
  Delay1 : Delay  DelayLength=double(1)  InitialCondition=0  SampleTime=1e-08
  Delay3 : Delay  DelayLength=double(1)  InitialCondition=0  SampleTime=1e-08
  Detect Fall Nonpositive : simulink/Logic and Bit Operations/Detect Fall Nonpositive  vinit=0  OutDataTypeStr=boolean
      settings: SourceProductBaseCode=SL
  Detect Rise Positive : simulink/Logic and Bit Operations/Detect Rise Positive  vinit=0  OutDataTypeStr=boolean
  Gain : Gain  Gain="fi(0,1,32,24,\"hex\",\"64000000\")"  ParamDataTypeStr=fixdt(1, 32, 24)  OutDataTypeStr=fixdt(1, 32, 24)  SampleTime=1e-08
  HDL Counter : hdlsllib/Sources/HDL Counter  CountType=Count limited  CountInit=double(1)  CountStep=double(1)  CountMax=double(2500000)  CountFromType=Initial value  CountFrom=double(1)  CountResetPort=on  CountLoadPort=off  CountEnbPort=off  CountDirPort=off  CountDataType=Unsigned  CountWordLen=32  CountFracLen=0  CountSampTime=1e-08
  HDL Reciprocal : Subsystem
  Product : Product  Inputs=**  OutDataTypeStr=fixdt(1, 32, 30)  SampleTime=1e-08
  Sum : Sum  Inputs=+-  AccumDataTypeStr=uint32  OutDataTypeStr=uint32  SampleTime=1e-08
  Switch : Switch  Criteria=u2 > Threshold  Threshold=double(0)  OutDataTypeStr=uint32  SampleTime=1e-08
  Switch1 : Switch  Criteria=u2 > Threshold  Threshold=double(0)  OutDataTypeStr=uint32  SampleTime=1e-08
  AXI_freq : Outport  VectorParamsAs1DForOutWhenUnconnected=off
  AXI_hightime : Outport  Port=2  VectorParamsAs1DForOutWhenUnconnected=off
  AXI_lowtime : Outport  Port=3  VectorParamsAs1DForOutWhenUnconnected=off
  AXI_dutycyc : Outport  Port=4  VectorParamsAs1DForOutWhenUnconnected=off
  wires:
  Delay3/1 -> Switch1/3
  Delay1/1 -> Switch/3
  Switch1/1 -> Delay3/1, AXI_hightime/1, Product/1, Sum/2
  Switch/1 -> Delay1/1, AXI_freq/1, HDL Reciprocal/1(In1), Sum/1
  Sum/1 -> AXI_lowtime/1
  Product/1 -> Gain/1
  HDL Reciprocal/1(Out1) -> Product/2
  HDL Counter/1 -> Delay/1, Compare To Constant1/1
  Gain/1 -> AXI_dutycyc/1
  Detect Rise Positive/1 -> HDL Counter/1
  Detect Fall Nonpositive/1 -> Compare To Constant/1
  Delay/1 -> Switch1/1, Switch/1
  Compare To Constant1/1 -> Switch/2
  Compare To Constant/1 -> Switch1/2
  PWMin/1 -> Detect Rise Positive/1, Detect Fall Nonpositive/1

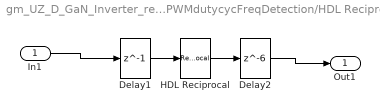
== system gm_UZ_D_GaN_Inverter_reduced/UZ_D_GaN_Inverter/PWMdutycycFreqDetection/HDL Reciprocal ==
  In1 : Inport
  Delay1 : Delay  DelayLength=1
  Delay2 : Delay  DelayLength=6
  HDL Reciprocal : Reciprocal  SampleTime=1e-08
  Out1 : Outport
  wires:
  In1/1 -> Delay1/1
  Delay1/1 -> HDL Reciprocal/1
  HDL Reciprocal/1 -> Delay2/1
  Delay2/1 -> Out1/1

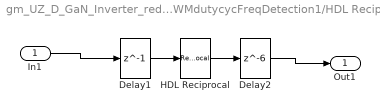
== system gm_UZ_D_GaN_Inverter_reduced/UZ_D_GaN_Inverter/PWMdutycycFreqDetection1/HDL Reciprocal ==
  In1 : Inport
  Delay1 : Delay  DelayLength=1
  Delay2 : Delay  DelayLength=6
  HDL Reciprocal : Reciprocal  SampleTime=1e-08
  Out1 : Outport
  wires:
  Delay2/1 -> Out1/1
  HDL Reciprocal/1 -> Delay2/1
  Delay1/1 -> HDL Reciprocal/1
  In1/1 -> Delay1/1

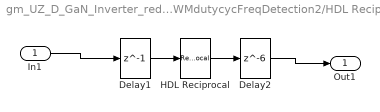
== system gm_UZ_D_GaN_Inverter_reduced/UZ_D_GaN_Inverter/PWMdutycycFreqDetection2/HDL Reciprocal ==
  In1 : Inport
  Delay1 : Delay  DelayLength=1
  Delay2 : Delay  DelayLength=6
  HDL Reciprocal : Reciprocal  SampleTime=1e-08
  Out1 : Outport
  wires:
  Delay2/1 -> Out1/1
  HDL Reciprocal/1 -> Delay2/1
  Delay1/1 -> HDL Reciprocal/1
  In1/1 -> Delay1/1

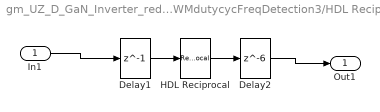
== system gm_UZ_D_GaN_Inverter_reduced/UZ_D_GaN_Inverter/PWMdutycycFreqDetection3/HDL Reciprocal ==
  In1 : Inport
  Delay1 : Delay  DelayLength=1
  Delay2 : Delay  DelayLength=6
  HDL Reciprocal : Reciprocal  SampleTime=1e-08
  Out1 : Outport
  wires:
  Delay2/1 -> Out1/1
  HDL Reciprocal/1 -> Delay2/1
  Delay1/1 -> HDL Reciprocal/1
  In1/1 -> Delay1/1

== system gm_UZ_D_GaN_Inverter_reduced/UZ_D_GaN_Inverter/PWMdutycycFreqDetection4/HDL Reciprocal ==
  In1 : Inport
  Delay1 : Delay  DelayLength=1
  Delay2 : Delay  DelayLength=6
  HDL Reciprocal : Reciprocal  SampleTime=1e-08
  Out1 : Outport
  wires:
  Delay2/1 -> Out1/1
  HDL Reciprocal/1 -> Delay2/1
  Delay1/1 -> HDL Reciprocal/1
  In1/1 -> Delay1/1

== system gm_UZ_D_GaN_Inverter_reduced/UZ_D_GaN_Inverter/PWMdutycycFreqDetection5/HDL Reciprocal ==
  In1 : Inport
  Delay1 : Delay  DelayLength=1
  Delay2 : Delay  DelayLength=6
  HDL Reciprocal : Reciprocal  SampleTime=1e-08
  Out1 : Outport
  wires:
  Delay2/1 -> Out1/1
  HDL Reciprocal/1 -> Delay2/1
  Delay1/1 -> HDL Reciprocal/1
  In1/1 -> Delay1/1
